simulink library "vmc"  (R2021b)
settings: Solver=VariableStepAuto  StartTime=0.0  StopTime=10.0  RelTol=1e-3
undefined symbols (not defined in the file or in its folder): AVMC_ACCDeltaTqIGain4OVRD_X_kph, AVMC_ACCDeltaTqIGain4OVRD_Y_mps2, AVMC_ACCDeltaTqIGain_X_kph, AVMC_ACCDeltaTqIGain_Y_mps2, AVMC_ACCDeltaTqPGain_X_kph, AVMC_ACCDeltaTqPGain_Y_kph, AVMC_ACCLongSteadyCtrl_X_kph, AVMC_ADSPosGFBDeltaTq_X_kph, AVMC_ADSPosGFBDeltaTq_Y_mps2, AVMC_AggressJerkPCT4AT_X_kph, AVMC_AggressJerkPCT_X_kph, AVMC_AggressLimitPCT4AT_X_kph, AVMC_AggressLimitPCT_X_kph, AVMC_CCLongSteadyCtrl_X_kph, AVMC_DISCDeltaTqIGain_X_kph, AVMC_DISCDeltaTqIGain_Y_mps2, AVMC_DISCDeltaTqPGain_X_kph, AVMC_DISCDeltaTqPGain_Y_kph, AVMC_ESCRegenOut_X_kph, AVMC_ESCRegenOut_Y_Deg, AVMC_ESCRegenOutEnSpd_X_Deg, AVMC_ISOAccLimit_X_mps, AVMC_ISODecLimit_X_mps, AVMC_ISOJerk_X_mps, AVMC_LatESCRegenOut_X_kph, AVMC_LatESCRegenOut_Y_Deg, AVMC_LongAccDeadZone_X_kph, AVMC_LongAccFiltTsforP2_X_Gps, AVMC_MCPresBaseTq_X_bar, AVMC_MSALongSteadyCtrl_X_kph, AVMC_MSAPedalOvrd_X_kph, AVMC_MSASpdBand_X_kph, AVMC_MSATqDownEndTq_X_kph, AVMC_MSATqDownTime_X_kph, AVMC_OPDDisSlideRate_X_Deg, AVMC_OVRD2ActSR2FCMCMD_X_mps2, AVMC_PedalTqRWhlRatio_X_Nm, AVMC_PedalTqRWhlRatio_Y_gps, AVMC_PedalTqRWhlSlipGain_X_rat, AVMC_PedalTqRWhlSlipGain_Y_kph, AVMC_PedalTqRWhSTRGGain_X_deg, AVMC_PedalTqRWhSTRGGain_Y_kph, AVMC_RDCDetectTime_X_kph, AVMC_RDCDetectTime_Y_pct, AVMC_RDCEnSlideRate_X_Deg, AVMC_RearWhlTqRatio_X_Nm, AVMC_RearWhlTqRatio_Y_gps, AVMC_RearWhlTqSlipGain_X_rat, AVMC_RearWhlTqSlipGain_Y_kph, AVMC_RearWhlTqSTRGGain_X_deg, AVMC_RearWhlTqSTRGGain_Y_kph, AVMC_ReqBrkJoinDecSR_X_mps2, AVMC_SoftJerkPCT_X_kph, AVMC_SoftLimitPCT_X_kph, AVMC_StESCYaw_X_kph, AVMC_StESCYaw_Y_Deg, AVMC_StESCYawCom_X_kph, AVMC_StESCYawCom_Y_Gps, AVMC_TMSpdBaseTq_X_rpm, AVMC_VehHoldDecCtrlTime2_X_kph ... (+411)
libraries: hcu_lib x108, simulink x82, tqr x1, simulink_extras x1
(part 9 of 14)

== system vmc/VMC/VMC/MSA function/MSAActivationHandshake ==
  VTQD_SpdCtrlMode_enum : Inport
  VVMC_FeatArbitrFinal_enum : Inport  Port=2
  VTQD_ExternalTqAllow_flg : Inport  Port=3
  VVMC_MeterIndSpeedForCalcu_kph : Inport  Port=4
  VVMC_FeatSetSpdFinal_raw32 : Inport  Port=5
  VTQD_SWC2CANCELSta_flg : Inport  Port=6
  VTQD_SWC2ResUpSta_flg : Inport  Port=7
  VTQD_SWC2SetdownSta_flg : Inport  Port=8
  VVMC_MSAOvrdAllow_flg : Inport  Port=9
  VINP_Distanceunit_flg : Inport  Port=10
  VTQD_GearActualPosn_enum : Inport  Port=11
  VVMC_VMCMSACtrlAvail_flg : Inport  Port=12
  VINP_SWCType_enum : Inport  Port=13
  VTQD_SWC1CANCELSta_flg : Inport  Port=14
  VTQD_SWC1ResUpSta_flg : Inport  Port=15
  VTQD_SWC1SetdownSta_flg : Inport  Port=16
  " 1" : Constant  Value=KTQD_MSAActiveMetSpdLoMPH_mph
  " 2" : Constant  Value=ENUM_SWCTYPE_SWC2
  " 80" : Constant  Value=KTQD_MSAActiveMetSpdLo_kph
  160 : Constant  Value=KTQD_MSAActiveMetSpdHi_kph
  2 : Constant  Value=KTQD_MSAActiveMetSpdHiMPH_mph
  AND : Logic  AllPortsSameDT=off  OutDataTypeStr=boolean
  AND1 : Logic  Operator=OR  AllPortsSameDT=off  OutDataTypeStr=boolean
  Cast To Boolean : DataTypeConversion  OutDataTypeStr=boolean
  Cast To Single : DataTypeConversion  OutDataTypeStr=uint8
  Cast To Single1 : DataTypeConversion  OutDataTypeStr=boolean
  Cast To Single2 : DataTypeConversion  OutDataTypeStr=single
  Cast To Single3 : DataTypeConversion  OutDataTypeStr=single
  Chart : Stateflow chart  TreatAsAtomicUnit=on
  Constant2 : Constant  Value=KVMC_CCMSASpdWar_kph
  Constant3 : Constant  Value=ENUM_ADASMSASTA_UNLIMIT
  Constant5 : Constant  Value=ENUM_FEATARBITRSTA_MSA
  Constant6 : Constant  Value=TRUE
  Constant7 : Constant  Value=FALSE
  Constant8 : Constant  Value=ENUM_ADASMSASTA_ACTIVE
  Detect Decrease2 : simulink/Logic and Bit Operations/Detect Decrease  vinit=0.0  OutDataTypeStr=boolean
  Detect Decrease3 : simulink/Logic and Bit Operations/Detect Decrease  vinit=0.0  OutDataTypeStr=boolean
  Detect Decrease4 : simulink/Logic and Bit Operations/Detect Decrease  vinit=0.0  OutDataTypeStr=boolean
  Detect Increase : simulink/Logic and Bit Operations/Detect Increase  vinit=0.0  OutDataTypeStr=boolean
  Detect Increase1 : simulink/Logic and Bit Operations/Detect Increase  vinit=0.0  OutDataTypeStr=boolean
  Detect Increase2 : simulink/Logic and Bit Operations/Detect Increase  vinit=0.0  OutDataTypeStr=boolean
  Relational Operator{,1..3} (4 alike) : RelationalOperator  Operator===  OutDataTypeStr=boolean  RndMeth=Simplest
  Switch{1..5} (5 alike) : Switch  Criteria=u2 > Threshold
  u2 > 0 : Switch  Criteria=u2 > Threshold
  VVMC_IntMSACtrlSta_enum : Outport
  VVMC_IntMSASpdWar_flg : Outport  Port=2
  VVMC_IntMSAActive_flg : Outport  Port=3
  wires:
  AND1/1 -> AND/2
  Relational Operator2/1 -> AND1/2
  Constant3/1 -> Relational Operator2/2
  [VVMC_IntMSACtrlSta_enum] -> Relational Operator2/1
  [VVMC_MSAOvrdAllow_flg] -> Chart/9(VVMC_MSAOvrdAllow_flg)
  VVMC_MSAOvrdAllow_flg/1 -> [VVMC_MSAOvrdAllow_flg]
  Cast To Single/1 -> [VVMC_IntMSACtrlSta_enum]  "VVMC_IntMSACtrlSta_enum"
  Cast To Boolean/1 -> [VVMC_IntMSAActive_flg]  "VVMC_IntMSAActive_flg"
  Cast To Single1/1 -> [VVMC_IntMSASpdWar_flg]  "VVMC_IntMSASpdWar_flg"
  VVMC_MeterIndSpeedForCalcu_kph/1 -> [VVMC_MeterIndSpeedForCalcu_kph]
  VVMC_FeatSetSpdFinal_raw32/1 -> [VVMC_FeatSetSpdFinal_raw32]
  VTQD_SWC2CANCELSta_flg/1 -> [VTQD_SWC2CANCELSta_flg]
  VTQD_ExternalTqAllow_flg/1 -> [VTQD_ExternalTqAllow_flg]
  VVMC_FeatArbitrFinal_enum/1 -> [VVMC_FeatArbitrFinal_enum]
  [VVMC_IntMSAActive_flg] -> VVMC_IntMSAActive_flg/1
  [VVMC_IntMSASpdWar_flg] -> VVMC_IntMSASpdWar_flg/1
  [VVMC_IntMSACtrlSta_enum] -> VVMC_IntMSACtrlSta_enum/1
  u2 > 0/1 -> Cast To Boolean/1
  Chart/2(VVMC_IntMSASpdWar_flg) -> Cast To Single1/1
  Chart/1(VVMC_IntMSACtrlSta_enum) -> Cast To Single/1
  Switch1/1 -> Chart/8(VVMC_DetectSWCCANCEL_flg)  "VVMC_DetectSWCCANCEL_flg"
  Constant2/1 -> Chart/7(KVMC_CCMSASpdWar_kph)
  [VVMC_FeatSetSpdFinal_raw32] -> Chart/6(VVMC_FeatSetSpdFinal_raw32)
  Switch3/1 -> Cast To Single3/1
  [VVMC_MeterIndSpeedForCalcu_kph] -> Chart/4(VVMC_MeterIndSpeedForCalcu_kph)
  Switch2/1 -> Cast To Single2/1
  [VTQD_ExternalTqAllow_flg] -> Chart/2(VTQD_ExternalTqAllow_flg)
  VTQD_SpdCtrlMode_enum/1 -> [VTQD_SpdCtrlMode_enum]
  [VTQD_SpdCtrlMode_enum] -> Chart/1(VTQD_SpdCtrlMode_enum)
  Constant8/1 -> Relational Operator1/2
  AND/1 -> u2 > 0/2
  [VVMC_FeatArbitrFinal_enum] -> Relational Operator/1
  Constant5/1 -> Relational Operator/2
  [VVMC_IntMSACtrlSta_enum] -> Relational Operator1/1
  Constant6/1 -> u2 > 0/1
  Relational Operator1/1 -> AND1/1
  Relational Operator/1 -> AND/1
  Constant7/1 -> u2 > 0/3
  Switch4/1 -> Chart/10(VVMC_DetectSWCRes_flg)  "VVMC_DetectSWCRes_flg"
  Switch5/1 -> Chart/11(VVMC_DetectSWCSet_flg)  "VVMC_DetectSWCSet_flg"
  VTQD_SWC2SetdownSta_flg/1 -> [VTQD_SWC2SetdownSta_flg]
  VTQD_SWC2ResUpSta_flg/1 -> [VTQD_SWC2ResUpSta_flg]
  [VINP_Distanceunit_flg] -> Switch2/2
  2/1 -> Switch2/1
  160/1 -> Switch2/3
  " 80"/1 -> Switch3/3
  " 1"/1 -> Switch3/1
  [VINP_Distanceunit_flg] -> Switch3/2
  VINP_Distanceunit_flg/1 -> [VINP_Distanceunit_flg]
  Cast To Single2/1 -> Chart/3(KVMC_MSAActiveMetSpdHi_kph)
  Cast To Single3/1 -> Chart/5(KVMC_MSAActiveMetSpdLo_kph)
  VTQD_GearActualPosn_enum/1 -> [VTQD_GearActualPosn_enum]
  [VTQD_GearActualPosn_enum] -> Chart/12(VTQD_GearActualPosn_enum)
  VVMC_VMCMSACtrlAvail_flg/1 -> [VVMC_VMCMSACtrlAvail_flg]
  [VVMC_VMCMSACtrlAvail_flg] -> Chart/13(VVMC_VMCMSACtrlAvail_flg)
  [VTQD_SWC2SetdownSta_flg] -> Detect Increase2/1
  [VINP_SWCType_enum] -> Relational Operator3/1
  " 2"/1 -> Relational Operator3/2
  [VTQD_SWC1SetdownSta_flg] -> Detect Decrease4/1
  Detect Increase1/1 -> Switch4/1
  [VTQD_SWC1ResUpSta_flg] -> Detect Decrease3/1
  Detect Decrease3/1 -> Switch4/3
  Detect Increase2/1 -> Switch5/1
  Detect Decrease2/1 -> Switch1/3
  [VTQD_SWC1CANCELSta_flg] -> Detect Decrease2/1
  [VTQD_SWC2CANCELSta_flg] -> Detect Increase/1
  Detect Increase/1 -> Switch1/1
  Relational Operator3/1 -> Switch5/2, Switch4/2, Switch1/2
  [VTQD_SWC2ResUpSta_flg] -> Detect Increase1/1
  Detect Decrease4/1 -> Switch5/3
  VINP_SWCType_enum/1 -> [VINP_SWCType_enum]
  VTQD_SWC1SetdownSta_flg/1 -> [VTQD_SWC1SetdownSta_flg]
  VTQD_SWC1ResUpSta_flg/1 -> [VTQD_SWC1ResUpSta_flg]
  VTQD_SWC1CANCELSta_flg/1 -> [VTQD_SWC1CANCELSta_flg]

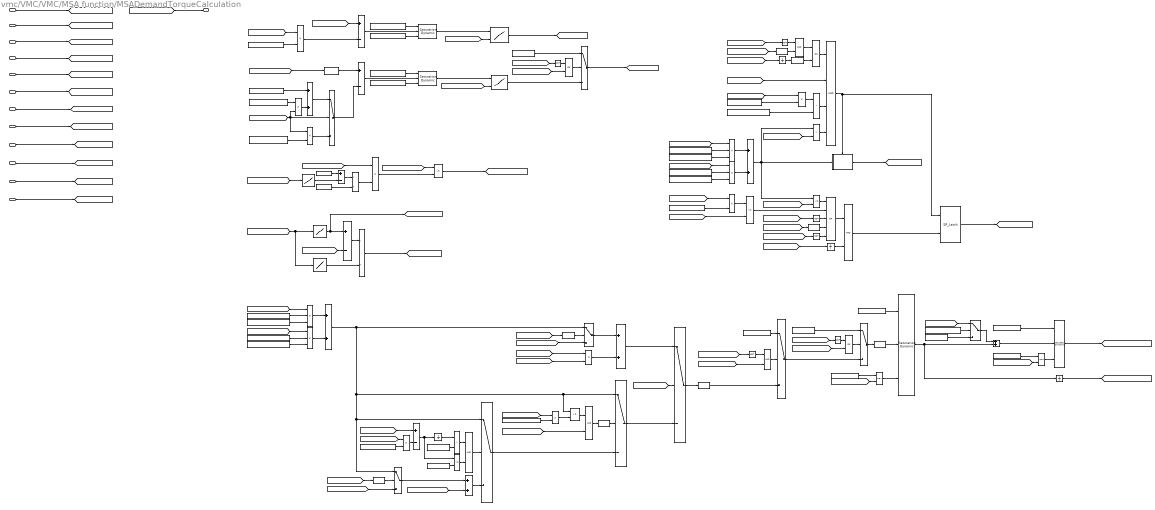
== system vmc/VMC/VMC/MSA function/MSADemandTorqueCalculation ==
  VVMC_FeatSetSpdForCalcu_kph : Inport
  VINP_VehSpeed_kph : Inport  Port=2
  VVMC_MSAActive_flg : Inport  Port=3
  VVMC_LongAcc_Gps : Inport  Port=4
  VVMC_MeterIndSpeedForCalcu_kph : Inport  Port=5
  VVMC_ActACCRequiredAccel_mps2 : Inport  Port=6
  VTQR_FrTMTqReq_Nm : Inport  Port=7
  VTQR_RrTMTqReq_Nm : Inport  Port=8
  VVMC_MSAPedalOvrd_flg : Inport  Port=9
  task_time_s : Inport  Port=10
  VTQD_LowIdleAccPedal_flg : Inport  Port=11
  VVMC_TotalAvailBrkRgnTq_Nm : Inport  Port=12
  1-D Lookup Table4 : Lookup_n-D  NumberOfTableDimensions=1  BreakpointsForDimension1=AVMC_MSASpdBand_X_kph  Table=MVMC_MSASpdBand_Y_pct  InternalRulePriority=Speed  RndMeth=Simplest  InputSameDT=on
  AND1 : Logic  Inputs=4  AllPortsSameDT=off  OutDataTypeStr=boolean
  AND2 : Logic  Operator=OR  Inputs=5  AllPortsSameDT=off  OutDataTypeStr=boolean
  AND{4..8} (5 alike) : Logic  AllPortsSameDT=off  OutDataTypeStr=boolean
  Add{,6,10,22..23} (5 alike) : Sum  Inputs=+-
  Add{1..3,5,8,12} (6 alike) : Sum
  Cast To Single4 : DataTypeConversion  OutDataTypeStr=single
  Cast To Single5 : DataTypeConversion  OutDataTypeStr=single
  Constant10 : Constant  Value=KVMC_MSATqUpLim_Nm  OutDataTypeStr=single
  Constant{18,20,31,107} (4 alike) : Constant  Value=KVMC_GravityValue_mps2
  Constant11 : Constant  Value=KVMC_MSATqUpLim_Nm  OutDataTypeStr=single
  Constant{6..7,12,41..42} (5 alike) : Constant  Value=ZERO_FLOAT
  Constant17 : Constant  Value=KVMC_MSAEnCtrlTargetAcc_mps2
  Constant2 : Constant  Value=pct
  Constant22 : Constant  Value=KTQD_RrTMTotalGearRatio_gain
  Constant23 : Constant  Value=KTQR_RrTMGearEff_c
  Constant24 : Constant  Value=KTQR_FrTMGearEff_c
  Constant25 : Constant  Value=KTQD_FrTMTotalGearRatio_gain
  Constant3 : Constant  Value=pct
  Constant32 : Constant  Value=KTQD_RrTMTotalGearRatio_gain
  Constant33 : Constant  Value=KTQR_RrTMGearEff_c
  Constant34 : Constant  Value=KTQR_FrTMGearEff_c
  Constant35 : Constant  Value=KTQD_FrTMTotalGearRatio_gain
  Constant36 : Constant  Value=KVMC_AccDevLowLim_mps2
  Constant38 : Constant  Value=KVMC_AccDevUpLim_mps2
  Constant39 : Constant  Value=KVMC_MSATqLowLim_Nm  OutDataTypeStr=single
  Constant4 : Constant  Value=KVMC_MSAPGainSW_flg
  Constant40 : Constant  Value=KVMC_MSASpdDevUpLim_kph
  Constant49 : Constant  Value=KVMC_MSATqUpLim_Nm  OutDataTypeStr=single
  Constant56 : Constant  Value=KVMC_MSASpdDevLowLim_kph
  Constant58 : Constant  Value=KVMC_Veh2MeterSpdFactor_enum
  Constant59 : Constant  Value=KVMC_Veh2MeterSpdOffset_enum
  Constant65 : Constant  Value=KVMC_Veh2MeterSpdLoFactor_enum
  Constant8 : Constant  Value=KVMC_MSATqLowLim_Nm  OutDataTypeStr=single
  Constant9 : Constant  Value=KVMC_MSATqDownEndTqRatio_pct
  Data Type Conversion1 : DataTypeConversion  OutDataTypeStr=single
  Detect Decrease1 : simulink/Logic and Bit Operations/Detect Decrease  vinit=0.0  OutDataTypeStr=boolean
  Detect Increase{,1..4} (5 alike) : simulink/Logic and Bit Operations/Detect Increase  vinit=0.0  OutDataTypeStr=boolean
  Divide : Product  Inputs=*/
  Divide{1..3,5} (4 alike) : Product  Inputs=***
  Divide{4,6,11..12} (4 alike) : Product  Inputs=**
  InitialCondition: 1 : UnitDelay  SampleTime=-1  HasFrameUpgradeWarning=on
  Logical Operator2 : Logic  Operator=OR  AllPortsSameDT=off  OutDataTypeStr=boolean
  MVMC_DISCDeltaTqIGain_Z_Nm : Lookup_n-D  BreakpointsForDimension1=AVMC_DISCDeltaTqIGain_Y_mps2  BreakpointsForDimension2=AVMC_DISCDeltaTqIGain_X_kph  Table=MVMC_DISCDeltaTqIGain_Z_Nm  InternalRulePriority=Speed  RndMeth=Simplest  InputSameDT=on
      settings: InputPortMap=u0,u1
  MVMC_DISCDeltaTqPGain_Z_Nm : Lookup_n-D  BreakpointsForDimension1=AVMC_DISCDeltaTqPGain_Y_kph  BreakpointsForDimension2=AVMC_DISCDeltaTqPGain_X_kph  BreakpointsForDimension3=[5, 7]  Table=MVMC_DISCDeltaTqPGain_Z_Nm  ExtrapMethod=Clip  InternalRulePriority=Speed  RndMeth=Simplest  InputSameDT=on
      settings: InputPortMap=u0,u1
  MVMC_MSATqDownEndTq_Y_Nm : Lookup_n-D  NumberOfTableDimensions=1  BreakpointsForDimension1=AVMC_MSATqDownEndTq_X_kph  Table=MVMC_MSATqDownEndTq_Y_Nm  InternalRulePriority=Speed  RndMeth=Simplest  InputSameDT=on
  MVMC_MSATqDownTime_Y_s : Lookup_n-D  NumberOfTableDimensions=1  BreakpointsForDimension1=AVMC_MSATqDownTime_X_kph  Table=MVMC_MSATqDownTime_Y_s  InternalRulePriority=Speed  RndMeth=Simplest  InputSameDT=on
  Max : MinMax  Function=max  Inputs=2
  Max1 : MinMax  Function=max  Inputs=2
  NOT{,1..5} (6 alike) : Logic  Operator=NOT  AllPortsSameDT=off  OutDataTypeStr=boolean
  OR : Logic  Operator=OR  AllPortsSameDT=off  OutDataTypeStr=boolean
  OR1 : Logic  Operator=OR  AllPortsSameDT=off  OutDataTypeStr=boolean
  Product{2..5,13} (5 alike) : Product
  Product14 : Product  Inputs=*/
  Relational Operator : RelationalOperator  Operator=>  OutDataTypeStr=boolean  RndMeth=Simplest
  Relational Operator1 : RelationalOperator  Operator=<=  OutDataTypeStr=boolean  RndMeth=Simplest
  Relational Operator10 : RelationalOperator  OutDataTypeStr=boolean  RndMeth=Simplest
  Relational Operator2 : RelationalOperator  Operator=>  OutDataTypeStr=boolean  RndMeth=Simplest
  Relational Operator3 : RelationalOperator  Operator=<=  OutDataTypeStr=boolean  RndMeth=Simplest
  Relational Operator4 : RelationalOperator  Operator=>  OutDataTypeStr=boolean  RndMeth=Simplest
  Relational Operator5 : RelationalOperator  Operator=<=  OutDataTypeStr=boolean  RndMeth=Simplest
  Relational Operator8 : RelationalOperator  OutDataTypeStr=boolean  RndMeth=Simplest
  SR_Latch5 : hcu_lib/Basic_Blocks/SR_Latch
  Saturation Dynamic{1,7..9} (4 alike) : simulink/Discontinuities/Saturation Dynamic  OutMin=[]  OutMax=[]  OutDataTypeStr=Inherit: Same as second input  OutDataType=fixdt(1, 16)  OutScaling=2^-10  DoSatur=off
  Switch{,2..6,8,10,12} (9 alike) : Switch  Criteria=u2 > Threshold
  Switch7 : Switch  Criteria=u2 > Threshold  Threshold=KVMC_Veh2MeterSpdLoBdy_kph
  Triggered Subsystem : Subsystem  TreatAsAtomicUnit=on
  Unit Delay : UnitDelay  SampleTime=-1  HasFrameUpgradeWarning=on
  Unit Delay2 : UnitDelay  SampleTime=-1  HasFrameUpgradeWarning=on
  Unit Delay3 : UnitDelay  SampleTime=-1  HasFrameUpgradeWarning=on
  VVMC_MSAWhlTqCal_Nm : Outport
  wires:
  [VVMC_MSAPedalOvrd_flg] -> NOT3/1
  NOT3/1 -> AND6/1
  AND6/1 -> Logical Operator2/1
  Unit Delay3/1 -> AND5/2
  [VVMC_MSATqDown_flg] -> Unit Delay3/1
  Detect Increase4/1 -> AND2/4
  NOT1/1 -> AND2/5
  [VVMC_MSAActive_flg] -> AND1/2
  AND4/1 -> Switch12/2
  Relational Operator4/1 -> AND4/1
  Relational Operator5/1 -> AND4/2
  Switch12/1 -> Switch4/3  "VVMC_MSAWhlTqCalAftGCtrl_Nm"
  Constant42/1 -> Relational Operator5/2
  Constant41/1 -> Relational Operator4/2
  Unit Delay/1 -> Relational Operator4/1
  Add10/1 -> Unit Delay/1, Relational Operator5/1
  [VVMC_LongAcc_Gps] -> Product5/1
  Constant31/1 -> Product5/2
  [VVMC_MSAReqAcc_mps2] -> Add10/1
  Product5/1 -> Add10/2
  VTQD_LowIdleAccPedal_flg/1 -> [VTQD_LowIdleAccPedal_flg]
  Relational Operator3/1 -> AND2/1
  [VVMC_MSATqDownEndTq_Nm] -> Relational Operator3/2
  [VVMC_MSAPedalOvrd_flg] -> Detect Increase4/1
  Switch/1 -> Add5/1
  [VVMC_LastMSAWhlTqCalW_Nm] -> Switch/3
  Detect Increase/1 -> Switch/2
  [VVMC_MSATqDown_flg] -> Detect Increase/1
  Logical Operator2/1 -> AND1/1
  Detect Decrease1/1 -> Logical Operator2/2
  [VVMC_MSAPedalOvrd_flg] -> Unit Delay2/1
  Unit Delay2/1 -> Detect Decrease1/1
  Divide6/1 -> Add5/2
  Add5/1 -> Switch10/1  "VVMC_MSAWhlTqCalAftTqDown_Nm"
  [task_time_s] -> Divide6/2
  [VVMC_MSATqDownSlope_Nmps] -> Divide6/1
  task_time_s/1 -> [task_time_s]
  Constant33/1 -> Divide5/3
  Divide3/1 -> Add2/1
  [VTQR_RrTMTqReq_Nm] -> Divide5/1
  Constant35/1 -> Divide3/2
  Constant32/1 -> Divide5/2
  Divide5/1 -> Add2/2
  Constant34/1 -> Divide3/3
  [VTQR_FrTMTqReq_Nm] -> Divide3/1
  [VVMC_MSATqDown_flg] -> Switch10/2
  Divide/1 -> [VVMC_MSATqDownSlope_Nmps]  "VVMC_MSATqDownSlope_Nmps"
  MVMC_MSATqDownTime_Y_s/1 -> Divide/2
  Add/1 -> Divide/1
  MVMC_MSATqDownEndTq_Y_Nm/1 -> [VVMC_MSATqDownEndTq_Nm], Add/1  "VVMC_MSATqDownEndTq_Nm"
  [VVMC_MSATqDownEnTq_Nm] -> Add/2
  [VVMC_MSATqDownEndTq_Nm] -> Relational Operator2/2
  Relational Operator2/1 -> AND1/4
  Triggered Subsystem/1(Out1) -> [VVMC_MSATqDownEnTq_Nm]  "VVMC_MSATqDownEnTq_Nm"
  SR_Latch5/1 -> [VVMC_MSATqDown_flg]  "VVMC_MSATqDown_flg"
  Relational Operator1/1 -> AND2/2
  NOT/1 -> AND2/3
  [VVMC_MSAActive_flg] -> NOT/1
  AND2/1 -> AND5/1
  Add1/1 -> Relational Operator3/1, Triggered Subsystem/1(In1), Relational Operator2/1
  [VTQR_FrTMTqReq_Nm] -> Divide1/1
  Constant24/1 -> Divide1/3
  Divide2/1 -> Add1/2
  Constant22/1 -> Divide2/2
  Constant25/1 -> Divide1/2
  [VTQR_RrTMTqReq_Nm] -> Divide2/1
  Constant23/1 -> Divide2/3
  Divide1/1 -> Add1/1
  AND1/1 -> SR_Latch5/1, Triggered Subsystem/Trigger
  Constant20/1 -> Product4/2
  [VVMC_LongAcc_Gps] -> Product4/1
  Product4/1 -> Relational Operator1/1
  [VVMC_MSAReqAcc_mps2] -> Relational Operator1/2
  Relational Operator/1 -> AND1/3
  Detect Increase2/1 -> AND6/2
  [VVMC_MSAInCtrlSpd_flg] -> Detect Increase2/1
  Constant17/1 -> Relational Operator/2
  Product3/1 -> Relational Operator/1
  [VVMC_LongAcc_Gps] -> Product3/1
  Constant18/1 -> Product3/2
  VVMC_MSAPedalOvrd_flg/1 -> [VVMC_MSAPedalOvrd_flg]
  VTQR_RrTMTqReq_Nm/1 -> [VTQR_RrTMTqReq_Nm]
  VTQR_FrTMTqReq_Nm/1 -> [VTQR_FrTMTqReq_Nm]
  VVMC_ActACCRequiredAccel_mps2/1 -> [VVMC_MSAReqAcc_mps2]
  [VVMC_FeatSetSpdForCalcu_kph] -> MVMC_DISCDeltaTqPGain_Z_Nm/2
  Switch3/1 -> Cast To Single5/1
  Saturation Dynamic9/1 -> MVMC_DISCDeltaTqPGain_Z_Nm/1
  [VVMC_MSAIGainDeltaTq_Nm] -> Add12/2
  InitialCondition: 1/1 -> [VVMC_LastMSAWhlTqCalW_Nm]  "VVMC_MSAWhlTqCalDelay_Nm"
  Add23/1 -> Saturation Dynamic9/2
  Switch6/1 -> Add12/1
  Saturation Dynamic8/1 -> MVMC_DISCDeltaTqIGain_Z_Nm/1
  Constant38/1 -> Saturation Dynamic8/1
  MVMC_DISCDeltaTqIGain_Z_Nm/1 -> [VVMC_MSAIGainDeltaTq_Nm]  "VVMC_MSAIGainDeltaTq_Nm"
  Data Type Conversion1/1 -> Add23/1
  Constant40/1 -> Saturation Dynamic9/1
  Saturation Dynamic7/1 -> InitialCondition: 1/1, Add3/2
  Add12/1 -> Switch12/3
  Constant39/1 -> Max/1
  Product2/1 -> Add22/2
  [VVMC_MSAReqAcc_mps2] -> Add22/1
  Constant107/1 -> Product2/2
  Cast To Single5/1 -> Saturation Dynamic7/2
  [VVMC_FeatSetSpdForCalcu_kph] -> Data Type Conversion1/1
  Constant36/1 -> Saturation Dynamic8/3
  [VINP_VehSpeed_kph] -> MVMC_DISCDeltaTqIGain_Z_Nm/2
  [VVMC_LongAcc_Gps] -> Product2/1
  Switch8/1 -> [VVMC_MSAPGainDeltaTq_Nm]  "VVMC_MSAPGainDeltaTq_Nm"
  Constant56/1 -> Saturation Dynamic9/3
  Switch10/1 -> Cast To Single4/1
  Add22/1 -> Saturation Dynamic8/2
  Constant49/1 -> Saturation Dynamic7/1
  VVMC_MeterIndSpeedForCalcu_kph/1 -> [VVMC_MeterIndSpeedForCalcu_kph]
  VVMC_LongAcc_Gps/1 -> [VVMC_LongAcc_Gps]
  VVMC_MSAActive_flg/1 -> [VVMC_MSAActive_flg]
  VINP_VehSpeed_kph/1 -> [VINP_VehSpeed_kph]
  VVMC_FeatSetSpdForCalcu_kph/1 -> [VVMC_FeatSetSpdForCalcu_kph]
  [VVMC_MSAWhlTqCal_Nm] -> VVMC_MSAWhlTqCal_Nm/1
  [VVMC_FeatSetSpdForCalcu_kph] -> MVMC_MSATqDownTime_Y_s/1, MVMC_MSATqDownEndTq_Y_Nm/1
  Cast To Single4/1 -> Switch5/3
  NOT4/1 -> OR/1
  [VTQD_LowIdleAccPedal_flg] -> AND7/2
  [VVMC_MSAInCtrlSpd_flg] -> AND8/2
  AND8/1 -> Detect Increase1/1
  Switch4/1 -> Switch10/3  "VVMC_MSAWhlTqCalNotTqDown_Nm"
  Add2/1 -> Switch/1, Switch6/1, Switch12/1, Relational Operator10/1, Switch4/1
  Relational Operator10/1 -> AND8/1
  [VVMC_MSATqDownEndTq_Nm] -> Divide4/1
  Detect Increase1/1 -> Switch4/2
  Divide4/1 -> Relational Operator10/2
  Constant9/1 -> Divide4/2
  [VVMC_MSAActive_flg] -> NOT4/1
  Constant6/1 -> Switch3/1
  OR/1 -> Switch3/2
  [VVMC_MSAPedalOvrd_flg] -> OR/2
  Switch5/1 -> Switch3/3  "VVMC_MSAWhlTqCalAftInCtrlSpd_Nm"
  AND7/1 -> Switch5/2
  Constant10/1 -> Switch5/1
  VVMC_TotalAvailBrkRgnTq_Nm/1 -> [VVMC_TotalAvailBrkRgnTq_Nm]
  [VVMC_TotalAvailBrkRgnTq_Nm] -> Max/2
  Max/1 -> Saturation Dynamic7/3
  [VVMC_MSAActive_flg] -> Detect Increase3/1
  Detect Increase3/1 -> Switch6/2
  [VVMC_LastMSAWhlTqCalW_Nm] -> Switch6/3
  [VVMC_FeatSetSpdForCalcu_kph] -> 1-D Lookup Table4/1
  [VVMC_MeterIndSpeedForCalcu_kph] -> Relational Operator8/1
  [VVMC_FeatSetSpdForCalcu_kph] -> Product13/1
  Constant2/1 -> Add6/1
  1-D Lookup Table4/1 -> Add6/2
  Add6/1 -> Product14/1
  Constant3/1 -> Product14/2
  Product14/1 -> Product13/2
  Product13/1 -> Relational Operator8/2
  Relational Operator8/1 -> [VVMC_MSAInCtrlSpd_flg]  "VVMC_MSAInCtrlSpd_flg"
  [VVMC_MSAInCtrlSpd_flg] -> NOT1/1
  [VVMC_MSAInCtrlSpd_flg] -> NOT2/1
  NOT2/1 -> AND7/1
  [VVMC_MSAPGainDeltaTq_Nm] -> Switch2/1
  Saturation Dynamic1/1 -> [VVMC_MSAWhlTqCal_Nm]  "VVMC_MSAWhlTqCal_Nm"
  Constant4/1 -> Switch2/2
  Constant7/1 -> Switch2/3
  Switch2/1 -> Add3/1
  Divide12/1 -> Switch7/3
  Constant65/1 -> Divide12/2
  Divide11/1 -> Add8/2
  Add8/1 -> Switch7/1
  Switch7/1 -> Add23/2
  Constant59/1 -> Add8/1
  Constant58/1 -> Divide11/1
  [VINP_VehSpeed_kph] -> Divide11/2, Switch7/2, Divide12/1
  Max1/1 -> Saturation Dynamic1/3
  [VVMC_TotalAvailBrkRgnTq_Nm] -> Max1/2
  Constant11/1 -> Saturation Dynamic1/1
  Constant8/1 -> Max1/1
  Add3/1 -> Saturation Dynamic1/2
  [VVMC_MSAPedalOvrd_flg] -> OR1/2
  OR1/1 -> Switch8/2
  Constant12/1 -> Switch8/1
  [VVMC_MSAActive_flg] -> NOT5/1
  NOT5/1 -> OR1/1
  MVMC_DISCDeltaTqPGain_Z_Nm/1 -> Switch8/3
  AND5/1 -> SR_Latch5/2

== system vmc/VMC/VMC/MSA function/MSATorqueSourceDetermination ==
  VVMC_MSAWhlTqCal_Nm : Inport
  VTQD_DriverWhlTqDem_Nm : Inport  Port=2
  VTQD_LowIdleAccPedal_flg : Inport  Port=3
  VDHP_ActAPSPosn_pct : Inport  Port=4
  VINP_VehSpeed_kph : Inport  Port=5
  task_time_s : Inport  Port=6
  VVMC_FeatSetSpdForCalcu_kph : Inport  Port=7
  VVMC_MeterIndSpeedForCalcu_kph : Inport  Port=8
  VVMC_MSAActive_flg : Inport  Port=9
  VTQD_SWCResUpSta_flg : Inport  Port=10
  VVMC_AntiSpdLimSpdEn_flg : Inport  Port=11
  1-D Lookup Table : Lookup_n-D  NumberOfTableDimensions=1  BreakpointsForDimension1=AVMC_MSASpdBand_X_kph  Table=MVMC_MSASpdBand_Y_pct  InternalRulePriority=Speed  RndMeth=Simplest  InputSameDT=on
  AND : Logic  Inputs=3  AllPortsSameDT=off  OutDataTypeStr=boolean
  Add11 : Sum  Inputs=+-
  Add2 : Sum
  Cast To Single5 : DataTypeConversion  OutDataTypeStr=single
  Constant : Constant  Value=KVMC_MSAOvrdJudgeSpd_kph
  Constant1 : Constant  Value=KVMC_MSAOvrdResAPSPosn_pct
  Constant10 : Constant  Value=TRUE
  Constant11 : Constant  Value=FALSE
  Constant13 : Constant  Value=KVMC_MSAOvrdTqRampSlope_Nmps
  Constant14 : Constant  Value=KVMC_MSATqLowLim_Nm  OutDataTypeStr=single
  Constant16 : Constant  Value=TRUE
  Constant17 : Constant  Value=FALSE
  Constant3 : Constant  Value=KVMC_MSAOvrdDetTime_s
  Constant4 : Constant  Value=KVMC_MSAOvrdResumeTime_s
  Constant43 : Constant  Value=pct
  Constant45 : Constant  Value=pct
  Constant49 : Constant  Value=KVMC_MSATqUpLim_Nm  OutDataTypeStr=single
  Detect Increase : simulink/Logic and Bit Operations/Detect Increase  vinit=0.0  OutDataTypeStr=boolean
  Detect Increase1 : simulink/Logic and Bit Operations/Detect Increase  vinit=0.0  OutDataTypeStr=boolean
  Detect Increase3 : simulink/Logic and Bit Operations/Detect Increase  vinit=0.0  OutDataTypeStr=boolean
  Divide : Product  Inputs=**
  Logical Operator : Logic  Inputs=3  AllPortsSameDT=off  OutDataTypeStr=boolean
  Logical Operator1 : Logic  Inputs=4  AllPortsSameDT=off  OutDataTypeStr=boolean
  Logical Operator2 : Logic  Operator=OR  AllPortsSameDT=off  OutDataTypeStr=boolean
  Logical Operator3 : Logic  Operator=OR  Inputs=3  AllPortsSameDT=off  OutDataTypeStr=boolean
  Logical Operator4 : Logic  Inputs=3  AllPortsSameDT=off  OutDataTypeStr=boolean
  Logical Operator5 : Logic  Operator=OR  AllPortsSameDT=off  OutDataTypeStr=boolean
  MVMC_MSAPedalOvrd_Y_pct1 : Lookup_n-D  NumberOfTableDimensions=1  BreakpointsForDimension1=AVMC_MSAPedalOvrd_X_kph  Table=MVMC_MSAPedalOvrd_Y_pct  ExtrapMethod=Clip  InternalRulePriority=Speed  RndMeth=Simplest  InputSameDT=on
  Min : MinMax  Inputs=2
  Min1 : MinMax  Inputs=2
  NOT{1..6} (6 alike) : Logic  Operator=NOT  AllPortsSameDT=off  OutDataTypeStr=boolean
  Product6 : Product
  Product7 : Product  Inputs=*/
  Relational Operator{,3,5..6} (4 alike) : RelationalOperator  OutDataTypeStr=boolean  RndMeth=Simplest
  Relational Operator1 : RelationalOperator  Operator=<=  OutDataTypeStr=boolean  RndMeth=Simplest
  Relational Operator2 : RelationalOperator  Operator=>  OutDataTypeStr=boolean  RndMeth=Simplest
  Relational Operator4 : RelationalOperator  Operator=<=  OutDataTypeStr=boolean  RndMeth=Simplest
  Relational Operator7 : RelationalOperator  Operator=>  OutDataTypeStr=boolean  RndMeth=Simplest
  Relational Operator8 : RelationalOperator  Operator=<=  OutDataTypeStr=boolean  RndMeth=Simplest
  SR_Latch1 : hcu_lib/Basic_Blocks/SR_Latch
  SR_Latch5 : hcu_lib/Basic_Blocks/SR_Latch
  Saturation Dynamic7 : simulink/Discontinuities/Saturation Dynamic  OutMin=[]  OutMax=[]  OutDataTypeStr=Inherit: Same as second input  OutDataType=fixdt(1, 16)  OutScaling=2^-10  DoSatur=off
  Switch : Switch  Criteria=u2 ~= 0
  Switch{1,3..6} (5 alike) : Switch  Criteria=u2 > Threshold
  Timer : hcu_lib/Basic_Blocks/Timer
  Timer1 : hcu_lib/Basic_Blocks/Timer
  Triggered Subsystem2 : Subsystem  TreatAsAtomicUnit=on
  Unit Delay{,1..3} (4 alike) : UnitDelay  SampleTime=-1  HasFrameUpgradeWarning=on
  VVMC_MSAWhlTqReq_Nm : Outport
  VVMC_MSAOvrdAllow_flg : Outport  Port=2
  VVMC_MSAWhlTqActive_flg : Outport  Port=3
  wires:
  Switch3/1 -> Switch1/2, Switch/2
  [VVMC_MSAWhlTqActive_flg] -> VVMC_MSAWhlTqActive_flg/1
  Switch1/1 -> [VVMC_MSAWhlTqActive_flg]  "VVMC_MSAWhlTqActive_flg"
  Constant10/1 -> Switch1/3
  Constant11/1 -> Switch1/1
  Relational Operator6/1 -> Logical Operator1/4
  Product6/1 -> Relational Operator6/2
  [VVMC_FeatSetSpdForCalcu_kph] -> Product6/1
  Constant45/1 -> Product7/2
  Product7/1 -> Product6/2
  [VVMC_MeterIndSpeedForCalcu_kph] -> Relational Operator6/1
  1-D Lookup Table/1 -> Add11/2
  Add11/1 -> Product7/1
  Constant43/1 -> Add11/1
  [VVMC_MSAActive_flg] -> NOT5/1
  NOT5/1 -> Logical Operator3/2
  [VVMC_MSAActive_flg] -> Logical Operator1/3
  NOT4/1 -> Logical Operator5/2
  [VVMC_MSAActive_flg] -> NOT4/1
  [VVMC_MSAActive_flg] -> Logical Operator/1
  VVMC_MSAActive_flg/1 -> [VVMC_MSAActive_flg]
  Timer1/1 -> Relational Operator5/1
  Constant4/1 -> Timer1/4, Relational Operator5/2
  [task_time_s] -> Timer1/3
  NOT3/1 -> Timer1/2
  [VVMC_MSAOvrdProhibit_flg] -> Logical Operator3/3
  Logical Operator3/1 -> Timer1/1, NOT3/1
  Logical Operator4/1 -> Logical Operator3/1
  VVMC_MeterIndSpeedForCalcu_kph/1 -> [VVMC_MeterIndSpeedForCalcu_kph]
  Detect Increase1/1 -> SR_Latch1/1, Triggered Subsystem2/Trigger
  Relational Operator3/1 -> Detect Increase1/1
  [VVMC_MSAOvrdAllow_flg] -> VVMC_MSAOvrdAllow_flg/1
  Timer/1 -> Relational Operator3/1
  VVMC_FeatSetSpdForCalcu_kph/1 -> [VVMC_FeatSetSpdForCalcu_kph]
  MVMC_MSAPedalOvrd_Y_pct1/1 -> Relational Operator7/2, Relational Operator2/2  "VVMC_MSAPedalOvrd_pct"
  [VVMC_MSAOvrdAllow_flg] -> Logical Operator2/1
  SR_Latch1/1 -> [VVMC_MSAOvrdAllow_flg]  "VVMC_MSAOvrdAllow_flg"
  Constant3/1 -> Timer/4, Relational Operator3/2
  [task_time_s] -> Timer/3
  task_time_s/1 -> [task_time_s]
  NOT2/1 -> Timer/2
  NOT1/1 -> Logical Operator1/2
  [VVMC_MSAOvrdProhibit_flg] -> NOT1/1
  Logical Operator1/1 -> Timer/1, NOT2/1
  [VDHP_ActAPSPosn_pct] -> Relational Operator2/1
  Switch6/1 -> [VVMC_MSAOvrdProhibit_flg]  "VVMC_MSAOvrdProhibit_flg"
  Detect Increase/1 -> Logical Operator5/1
  [VTQD_LowIdleAccPedal_flg] -> Detect Increase/1
  Relational Operator7/1 -> Logical Operator/2
  Relational Operator1/1 -> Logical Operator/3
  Constant/1 -> Relational Operator1/2
  [VINP_VehSpeed_kph] -> Relational Operator1/1
  VINP_VehSpeed_kph/1 -> [VINP_VehSpeed_kph]
  VDHP_ActAPSPosn_pct/1 -> [VDHP_ActAPSPosn_pct]
  VTQD_LowIdleAccPedal_flg/1 -> [VTQD_LowIdleAccPedal_flg]
  VTQD_DriverWhlTqDem_Nm/1 -> [VTQD_DriverWhlTqDem_Nm]
  VVMC_MSAWhlTqCal_Nm/1 -> [VVMC_MSAWhlTqCal_Nm]
  [VVMC_MSAWhlTqReq_Nm] -> VVMC_MSAWhlTqReq_Nm/1
  Switch/1 -> [VVMC_MSAWhlTqReq_Nm], Unit Delay1/1  "VVMC_MSAWhlTqReq_Nm"
  [VVMC_MSAWhlTqCal_Nm] -> Min1/1
  [VTQD_DriverWhlTqDem_Nm] -> Relational Operator/2
  Relational Operator/1 -> Logical Operator2/2
  [VVMC_MSAWhlTqCal_Nm] -> Relational Operator/1
  [VTQD_DriverWhlTqDem_Nm] -> Switch4/3
  VTQD_SWCResUpSta_flg/1 -> [VTQD_SWCResUpSta_flg]
  [VVMC_MSAWhlTqActive_flg] -> Unit Delay/1
  Unit Delay/1 -> AND/1
  [VTQD_SWCResUpSta_flg] -> AND/2
  AND/1 -> Switch3/2
  Constant17/1 -> Switch3/1
  Logical Operator2/1 -> Switch3/3
  [VVMC_FeatSetSpdForCalcu_kph] -> 1-D Lookup Table/1
  NOT6/1 -> AND/3
  [VTQD_LowIdleAccPedal_flg] -> NOT6/1
  Relational Operator2/1 -> Logical Operator1/1
  Unit Delay1/1 -> [VVMC_LastMSAWhlTqReq_Nm]
  Switch4/1 -> Switch/1
  [VVMC_MSAOvrdEnTq_Nm] -> Switch5/1
  Constant13/1 -> Divide/1
  [task_time_s] -> Divide/2
  Divide/1 -> Add2/2
  Constant14/1 -> Saturation Dynamic7/3
  Add2/1 -> Cast To Single5/1
  Constant49/1 -> Saturation Dynamic7/1
  Cast To Single5/1 -> Saturation Dynamic7/2
  Saturation Dynamic7/1 -> Min/1, Unit Delay2/1  "VVMC_MSAOvrdWhlTqCal_Nm"
  [VTQD_DriverWhlTqDem_Nm] -> Min/2
  Min/1 -> Switch4/1
  [VVMC_LastMSAWhlTqReq_Nm] -> Triggered Subsystem2/1(In1)
  Triggered Subsystem2/1(Out1) -> [VVMC_MSAOvrdEnTq_Nm]  "VVMC_MSAOvrdEnTq_Nm"
  [VVMC_MSAOvrdAllow_flg] -> Detect Increase3/1
  Detect Increase3/1 -> Switch5/2
  Switch5/1 -> Add2/1
  Unit Delay2/1 -> Switch5/3
  [VVMC_MSAOvrdAllow_flg] -> Switch4/2
  VVMC_AntiSpdLimSpdEn_flg/1 -> [VVMC_AntiSpdLimSpdEn_flg]
  [VVMC_AntiSpdLimSpdEn_flg] -> Switch6/2
  SR_Latch5/1 -> Switch6/3
  Constant16/1 -> Switch6/1
  Logical Operator5/1 -> SR_Latch5/2
  Logical Operator/1 -> SR_Latch5/1
  Min1/1 -> Switch/3
  [VTQD_DriverWhlTqDem_Nm] -> Min1/2
  Relational Operator5/1 -> SR_Latch1/2
  [VDHP_ActAPSPosn_pct] -> Relational Operator7/1
  [VVMC_FeatSetSpdForCalcu_kph] -> MVMC_MSAPedalOvrd_Y_pct1/1
  [VVMC_MSAOvrdAllow_flg] -> Unit Delay3/1
  Relational Operator4/1 -> Logical Operator4/2
  Unit Delay3/1 -> Logical Operator4/1
  [VVMC_MeterIndSpeedForCalcu_kph] -> Relational Operator8/1
  [VVMC_FeatSetSpdForCalcu_kph] -> Relational Operator8/2
  Relational Operator8/1 -> Logical Operator4/3
  [VDHP_ActAPSPosn_pct] -> Relational Operator4/1
  Constant1/1 -> Relational Operator4/2

== system vmc/VMC/VMC/RDC Determination/RWD ==
  task_time_s : Inport
  VVMC_ActMaxSlideRate_pct : Inport  Port=2
  VTQD_AfterAvailableTqDemFr_Nm : Inport  Port=3
  VTQD_AfterAvailableTqDemRr_Nm : Inport  Port=4
  VINP_ESCActive_flg : Inport  Port=5
  VINP_SASAngle_Deg : Inport  Port=6
  VINP_LatAccel_Gps : Inport  Port=7
  VINP_VehSpeed_kph : Inport  Port=8
  VINP_YawRate_degps : Inport  Port=9
  VINP_RDCActive_enum : Inport  Port=10
  VINP_DIDGetDynoMode_flg : Inport  Port=11
  AND{,2..5} (5 alike) : Logic  AllPortsSameDT=off  OutDataTypeStr=boolean
  AND1 : Logic  Inputs=3  AllPortsSameDT=off  OutDataTypeStr=boolean
  Abs{,1..7} (8 alike) : Abs
  Add1 : Sum
  Constant1 : Constant  Value=ZERO_INT
  Constant2 : Constant  Value=KVMC_DIDGetDynoModeSW_flg
  Constant{3..4,74,78} (4 alike) : Constant  Value=KVMC_AltRDCActiveTq_Nm
  Constant73 : Constant  Value=ENUM_RDCACTSTA_NOREQUEST
  Constant77 : Constant  Value=ENUM_RDCACTSTA_RAMPOUT
  Constant81 : Constant  Value=KVMC_AltRDCActiveSW_flg
  Constant82 : Constant  Value=ENUM_RDCACTSTA_EXITIMMEDIATELY
  Constant83 : Constant  Value=KVMC_AltRDCRecTime_s
  Constant86 : Constant  Value=KVMC_ESCRegenTqRecDelay_s
  Constant95 : Constant  Value=ENUM_RDCACTSTA_EXITIMMEDIATELY
  Delay{1..2,6..7} (4 alike) : Delay  DelayLength=1
  DelayEnable1 : hcu_lib/Basic_Blocks/DelayEnable
  DelayEnable2 : hcu_lib/Basic_Blocks/DelayEnable
  DelayEnable3 : hcu_lib/Basic_Blocks/DelayEnable
  Equal33 : RelationalOperator  Operator===  OutDataTypeStr=boolean  RndMeth=Simplest
  MVMC_ESCRegenOutEnSpd_Y_kph : Lookup_n-D  NumberOfTableDimensions=1  BreakpointsForDimension1=AVMC_ESCRegenOutEnSpd_X_Deg  Table=MVMC_ESCRegenOutEnSpd_Y_kph  ExtrapMethod=Clip  InternalRulePriority=Speed  RndMeth=Simplest  InputSameDT=on
  MVMC_ESCRegenOut_Z_Dps : Lookup_n-D  BreakpointsForDimension1=AVMC_ESCRegenOut_Y_Deg  BreakpointsForDimension2=AVMC_ESCRegenOut_X_kph  Table=MVMC_ESCRegenOut_Z_Dps  ExtrapMethod=Clip  InternalRulePriority=Speed  RndMeth=Simplest  InputSameDT=on
      settings: InputPortMap=u0,u1
  MVMC_LatESCRegenOut_Z_Gps : Lookup_n-D  BreakpointsForDimension1=AVMC_LatESCRegenOut_Y_Deg  BreakpointsForDimension2=AVMC_LatESCRegenOut_X_kph  Table=MVMC_LatESCRegenOut_Z_Gps  ExtrapMethod=Clip  InternalRulePriority=Speed  RndMeth=Simplest  InputSameDT=on
      settings: InputPortMap=u0,u1
  MVMC_RDCDetectTime_Z_s : Lookup_n-D  BreakpointsForDimension1=AVMC_RDCDetectTime_Y_pct  BreakpointsForDimension2=AVMC_RDCDetectTime_X_kph  Table=MVMC_RDCDetectTime_Z_s  ExtrapMethod=Clip  InternalRulePriority=Speed  RndMeth=Simplest  InputSameDT=on
      settings: InputPortMap=u0,u1
  MVMC_RDCEnSlideRate_Y_pct : Lookup_n-D  NumberOfTableDimensions=1  BreakpointsForDimension1=AVMC_RDCEnSlideRate_X_Deg  Table=MVMC_RDCEnSlideRate_Y_pct  ExtrapMethod=Clip  InternalRulePriority=Speed  RndMeth=Simplest  InputSameDT=on
  MVMC_StESCYawCom_Z_Dps : Lookup_n-D  BreakpointsForDimension1=AVMC_StESCYawCom_Y_Gps  BreakpointsForDimension2=AVMC_StESCYawCom_X_kph  Table=MVMC_StESCYawCom_Z_Dps  ExtrapMethod=Clip  InternalRulePriority=Speed  RndMeth=Simplest  InputSameDT=on
      settings: InputPortMap=u0,u1
  MVMC_StESCYaw_Z_Dps : Lookup_n-D  BreakpointsForDimension1=AVMC_StESCYaw_Y_Deg  BreakpointsForDimension2=AVMC_StESCYaw_X_kph  Table=MVMC_StESCYaw_Z_Dps  ExtrapMethod=Clip  InternalRulePriority=Speed  RndMeth=Simplest  InputSameDT=on
      settings: InputPortMap=u0,u1
  NOT : Logic  Operator=NOT  AllPortsSameDT=off  OutDataTypeStr=boolean
  NOT1 : Logic  Operator=NOT  AllPortsSameDT=off  OutDataTypeStr=boolean
  NOT3 : Logic  Operator=NOT  AllPortsSameDT=off  OutDataTypeStr=boolean
  OR{,1..4,9} (6 alike) : Logic  Operator=OR  AllPortsSameDT=off  OutDataTypeStr=boolean
  OR8 : Logic  AllPortsSameDT=off  OutDataTypeStr=boolean
  Relational Operator{1,8..10} (4 alike) : RelationalOperator  OutDataTypeStr=boolean  RndMeth=Simplest
  Relational Operator{2..7} (6 alike) : RelationalOperator  Operator=<=  OutDataTypeStr=boolean  RndMeth=Simplest
  SR_Latch4 : hcu_lib/Basic_Blocks/SR_Latch
  SR_Latch5 : hcu_lib/Basic_Blocks/SR_Latch
  Switch10 : Switch  Criteria=u2 > Threshold
  Switch11 : Switch  Criteria=u2 > Threshold
  Switch8 : Switch  Criteria=u2 > Threshold
  VVMC_RWDRDCActive_enum : Outport
  VVMC_RDCEnSlideRate_pct : Outport  Port=2
  VVMC_ActStESCYaw_Dps : Outport  Port=3
  wires:
  [VVMC_RDCDetectTime_s] -> DelayEnable1/2
  MVMC_RDCEnSlideRate_Y_pct/1 -> VVMC_RDCEnSlideRate_pct/1, [VVMC_RDCEnSlideRate_pct]  "VVMC_RDCEnSlideRate_pct"
  VINP_YawRate_degps/1 -> [VINP_YawRate_degps]
  [VINP_ESCActive_flg] -> NOT1/1
  VINP_ESCActive_flg/1 -> [VINP_ESCActive_flg]
  OR2/1 -> AND3/1
  Constant73/1 -> Switch8/3
  Delay7/1 -> Relational Operator3/1
  VINP_LatAccel_Gps/1 -> [VINP_LatAccel_Gps]
  [VVMC_RDCEnSlideRate_pct] -> Relational Operator1/2
  Switch11/1 -> [VVMC_AltRDCActive_enum]  "VVMC_AltRDCActive_enum"
  VINP_VehSpeed_kph/1 -> [VINP_VehSpeed_kph]
  Constant78/1 -> Relational Operator3/2
  [VINP_SASAngle_Deg] -> Abs7/1
  VVMC_ActMaxSlideRate_pct/1 -> [VVMC_ActMaxSlideRate_pct]
  DelayEnable2/1 -> OR3/2  "VVMC_AltRDCRec_flg"
  [task_time_s] -> DelayEnable1/3
  OR9/1 -> AND4/1
  [VINP_SASAngle_Deg] -> MVMC_LatESCRegenOut_Z_Gps/1
  [VVMC_ActMaxSlideRate_pct] -> MVMC_RDCDetectTime_Z_s/1
  [VINP_LatAccel_Gps] -> Abs5/1
  VTQD_AfterAvailableTqDemRr_Nm/1 -> [VTQD_AfterAvailableTqDemRr_Nm]
  SR_Latch5/1 -> [VVMC_ESCActive_flg]  "VVMC_ESCActive_flg"
  Abs4/1 -> Relational Operator8/1
  DelayEnable1/1 -> SR_Latch4/1  "VVMC_RDCDetectEn_flg"
  Relational Operator8/1 -> OR9/2
  Constant74/1 -> Relational Operator2/2
  [VVMC_ESCSlip_flg] -> SR_Latch5/1
  Abs5/1 -> Relational Operator10/1
  [VINP_SASAngle_Deg] -> MVMC_ESCRegenOut_Z_Dps/1
  [VINP_VehSpeed_kph] -> Relational Operator9/1
  Switch8/1 -> Switch11/3
  NOT3/1 -> OR8/1
  [VTQD_AfterAvailableTqDemFr_Nm] -> Delay6/1
  Delay6/1 -> Relational Operator2/1
  MVMC_RDCDetectTime_Z_s/1 -> [VVMC_RDCDetectTime_s]  "VVMC_RDCDetectTime_s"
  [VTQD_AfterAvailableTqDemRr_Nm] -> Delay7/1
  [VINP_SASAngle_Deg] -> MVMC_RDCEnSlideRate_Y_pct/1
  AND3/1 -> DelayEnable1/1
  [VVMC_ESCActive_flg] -> OR4/1
  Relational Operator3/1 -> OR2/2
  Relational Operator9/1 -> AND4/2, AND1/1
  Relational Operator1/1 -> AND3/2
  MVMC_ESCRegenOut_Z_Dps/1 -> Relational Operator8/2  "VVMC_ESCRegenOut_Dps"
  [VINP_YawRate_degps] -> Abs4/1
  SR_Latch4/1 -> Switch8/2
  [VVMC_ActMaxSlideRate_pct] -> Abs2/1
  Switch10/1 -> VVMC_RWDRDCActive_enum/1  "VVMC_RWDRDCActive_enum"
  [VINP_RDCActive_enum] -> Equal33/1
  VINP_SASAngle_Deg/1 -> [VINP_SASAngle_Deg]
  [task_time_s] -> DelayEnable3/3
  Abs2/1 -> Relational Operator1/1
  MVMC_LatESCRegenOut_Z_Gps/1 -> Relational Operator10/2  "VVMC_LatESCRegenOut_Gps"
  NOT1/1 -> OR8/2
  Equal33/1 -> OR4/2
  [VINP_VehSpeed_kph] -> MVMC_LatESCRegenOut_Z_Gps/2
  [VVMC_ESCSlip_flg] -> NOT3/1
  Relational Operator2/1 -> OR2/1
  Relational Operator10/1 -> OR9/1
  Constant95/1 -> Switch11/1
  [VINP_VehSpeed_kph] -> MVMC_ESCRegenOut_Z_Dps/2
  OR8/1 -> DelayEnable3/1
  OR4/1 -> Switch11/2
  [VVMC_AltRDCActive_enum] -> Switch10/1
  DelayEnable3/1 -> SR_Latch5/2
  Constant77/1 -> Switch8/1
  Constant86/1 -> DelayEnable3/2
  Constant82/1 -> Equal33/2
  VTQD_AfterAvailableTqDemFr_Nm/1 -> [VTQD_AfterAvailableTqDemFr_Nm]
  VINP_RDCActive_enum/1 -> [VINP_RDCActive_enum]
  task_time_s/1 -> [task_time_s]
  Constant1/1 -> Switch10/3
  [VINP_LatAccel_Gps] -> Abs1/1
  [VINP_SASAngle_Deg] -> Abs/1
  Abs/1 -> MVMC_StESCYaw_Z_Dps/1
  Add1/1 -> VVMC_ActStESCYaw_Dps/1, [VVMC_ActStESCYaw_Dps]  "VVMC_ActStESCYaw_Dps"
  MVMC_StESCYaw_Z_Dps/1 -> Add1/1  "VVMC_StESCYaw_Dps"
  [VINP_VehSpeed_kph] -> MVMC_StESCYaw_Z_Dps/2
  [VINP_VehSpeed_kph] -> MVMC_StESCYawCom_Z_Dps/2
  MVMC_StESCYawCom_Z_Dps/1 -> Add1/2  "VVMC_StESCYawCom_Dps"
  Abs1/1 -> MVMC_StESCYawCom_Z_Dps/1
  [VINP_VehSpeed_kph] -> MVMC_RDCDetectTime_Z_s/2
  AND/1 -> DelayEnable2/1
  [task_time_s] -> DelayEnable2/3
  Relational Operator4/1 -> AND/1
  [VVMC_ActStESCYaw_Dps] -> Relational Operator6/2
  [VVMC_RDCEnSlideRate_pct] -> Relational Operator4/2
  Abs6/1 -> Relational Operator6/1
  Relational Operator6/1 -> AND/2
  Abs3/1 -> Relational Operator4/1
  [VVMC_ActMaxSlideRate_pct] -> Abs3/1
  Constant83/1 -> DelayEnable2/2
  [VINP_YawRate_degps] -> Abs6/1
  Abs7/1 -> MVMC_ESCRegenOutEnSpd_Y_kph/1
  MVMC_ESCRegenOutEnSpd_Y_kph/1 -> Relational Operator9/2  "VVMC_ESCRegenOutEnSpd_kph"
  Constant4/1 -> Relational Operator7/2
  Delay1/1 -> Relational Operator5/1
  [VTQD_AfterAvailableTqDemRr_Nm] -> Delay2/1
  Constant3/1 -> Relational Operator5/2
  Delay2/1 -> Relational Operator7/1
  Relational Operator7/1 -> OR1/2
  Relational Operator5/1 -> OR1/1
  [VTQD_AfterAvailableTqDemFr_Nm] -> Delay1/1
  OR1/1 -> AND1/3
  [VINP_ESCActive_flg] -> AND1/2
  AND4/1 -> OR/1
  AND1/1 -> OR/2
  OR/1 -> [VVMC_ESCSlip_flg]  "VVMC_ESCSlip_flg"
  Constant81/1 -> AND2/1
  AND2/1 -> Switch10/2
  VINP_DIDGetDynoMode_flg/1 -> [VINP_DIDGetDynoMode_flg]
  [VINP_DIDGetDynoMode_flg] -> AND5/1
  Constant2/1 -> AND5/2
  AND5/1 -> NOT/1
  NOT/1 -> AND2/2
  [VINP_ESCActive_flg] -> OR3/1
  OR3/1 -> SR_Latch4/2

== system vmc/VMC/VMC/SPD2ACC/ISO22179 ==
  VVMC_VehSpeed_mps : Inport
  VVMC_LimitPCT_pct : Inport  Port=2
  VDSC_PreACC_flg : Inport  Port=3
  VDSC_DISCSta_enum : Inport  Port=4
  VDSC_AutoTurnMode_flg : Inport  Port=5
  VDSC_AccDecResp_flg : Inport  Port=6
  AND : Logic  AllPortsSameDT=off  OutDataTypeStr=boolean
  AND1 : Logic  Inputs=3  AllPortsSameDT=off  OutDataTypeStr=boolean
  AND2 : Logic  Inputs=3  AllPortsSameDT=off  OutDataTypeStr=boolean
  AND3 : Logic  Inputs=3  AllPortsSameDT=off  OutDataTypeStr=boolean
  Constant : Constant  Value=pct
  Constant1 : Constant  Value=MINUSONE_FLOAT
  Constant2 : Constant  Value=KVMC_DISCDecCtrlTest_flg
  Constant3 : Constant  Value=ENUM_DISCSTA_ACTIVE
  Constant4 : Constant  Value=KVMC_DISCDecCtrlJerk_mps3
  Constant5 : Constant  Value=KVMC_AutoTurnLimitHiGain_pct
  Constant6 : Constant  Value=KVMC_AutoTurnJerkHiGain_pct
  Constant7 : Constant  Value=KVMC_DISCDecCtrlLimit_mps2
  Constant8 : Constant  Value=KVMC_AutoTurnLimitHiGain_pct
  Constant9 : Constant  Value=KVMC_DISCAccCtrlLimit_mps2
  Divide{,1,3..6} (6 alike) : Product  Inputs=**
  Divide2 : Product  Inputs=*/
  MVMC_ISOAccLimit_Y_mps2 : Lookup_n-D  NumberOfTableDimensions=1  BreakpointsForDimension1=AVMC_ISOAccLimit_X_mps  UseOneInputPortForAllInputData=on  Table=MVMC_ISOAccLimit_Y_mps2  UseLastTableValue=on  InternalRulePriority=Speed  RndMeth=Simplest  InputSameDT=on
  MVMC_ISODecLimit_Y_mps2 : Lookup_n-D  NumberOfTableDimensions=1  BreakpointsForDimension1=AVMC_ISODecLimit_X_mps  UseOneInputPortForAllInputData=on  Table=MVMC_ISODecLimit_Y_mps2  UseLastTableValue=on  InternalRulePriority=Speed  RndMeth=Simplest  InputSameDT=on
  MVMC_ISOJerk_Y_mps3 : Lookup_n-D  NumberOfTableDimensions=1  BreakpointsForDimension1=AVMC_ISOJerk_X_mps  UseOneInputPortForAllInputData=on  Table=MVMC_ISOJerk_Y_mps3  UseLastTableValue=on  InternalRulePriority=Speed  RndMeth=Simplest  InputSameDT=on
  OR : Logic  Operator=OR  Inputs=3  AllPortsSameDT=off  OutDataTypeStr=boolean
  Relational Operator : RelationalOperator  Operator===  OutDataTypeStr=boolean  RndMeth=Simplest
  Switch{,1..5} (6 alike) : Switch  Criteria=u2 > Threshold
  VVMC_ISOAccLimit_mps2 : Outport
  VVMC_ISODecLimit_mps2 : Outport  Port=2
  VVMC_ISOJerkLimit_mps3 : Outport  Port=3
  wires:
  Constant1/1 -> Divide3/1
  [VVMC_ISOJerkLimit_mps3] -> VVMC_ISOJerkLimit_mps3/1  "VVMC_ISOJerkLimit_mps3"
  [VVMC_ISODecLimit_mps2] -> VVMC_ISODecLimit_mps2/1  "VVMC_ISODecLimit_mps2"
  [VVMC_ISOAccLimit_mps2] -> VVMC_ISOAccLimit_mps2/1  "VVMC_ISOAccLimit_mps2"
  [VVMC_VehSpeed_mps] -> MVMC_ISOJerk_Y_mps3/1
  Constant/1 -> Divide2/2
  [VVMC_LimitPCT_pct] -> Divide2/1
  VVMC_LimitPCT_pct/1 -> [VVMC_LimitPCT_pct]
  VVMC_VehSpeed_mps/1 -> [VVMC_VehSpeed_mps]
  Divide/1 -> Switch2/3
  MVMC_ISOJerk_Y_mps3/1 -> Switch/3
  MVMC_ISOAccLimit_Y_mps2/1 -> Divide/2
  [VVMC_VehSpeed_mps] -> MVMC_ISODecLimit_Y_mps2/1
  Divide3/1 -> Divide1/1
  Divide2/1 -> Divide/1, Divide1/2
  MVMC_ISODecLimit_Y_mps2/1 -> Divide3/2
  [VVMC_VehSpeed_mps] -> MVMC_ISOAccLimit_Y_mps2/1
  VDSC_AccDecResp_flg/1 -> [VDSC_AccDecResp_flg]
  VDSC_PreACC_flg/1 -> [VDSC_PreACC_flg]
  VDSC_AutoTurnMode_flg/1 -> [VDSC_AutoTurnMode_flg]
  VDSC_DISCSta_enum/1 -> [VDSC_DISCSta_enum]
  Constant5/1 -> Divide5/1
  Switch1/1 -> Divide5/2, Switch4/3
  [VDSC_AccDecResp_flg] -> AND3/1
  Divide5/1 -> Switch4/1
  [VDSC_AutoTurnMode_flg] -> AND3/2
  AND3/1 -> Switch4/2
  Constant7/1 -> Switch1/1
  Divide1/1 -> Switch1/3
  [VVMC_DISCDecCtrl_flg] -> AND3/3
  [VVMC_DISCDecCtrl_flg] -> Switch1/2
  Switch4/1 -> [VVMC_ISODecLimit_mps2]
  [VVMC_DISCDecCtrl_flg] -> AND2/3
  [VDSC_AccDecResp_flg] -> AND2/1
  Constant2/1 -> AND/2
  Relational Operator/1 -> OR/2
  AND2/1 -> Switch3/2
  [VDSC_AutoTurnMode_flg] -> AND2/2
  Switch/1 -> Divide4/2, Switch3/3
  [VDSC_DISCSta_enum] -> Relational Operator/1
  Constant3/1 -> Relational Operator/2
  Divide4/1 -> Switch3/1
  Constant6/1 -> Divide4/1
  OR/1 -> AND/1
  [VDSC_AutoTurnMode_flg] -> OR/3
  Constant4/1 -> Switch/1
  AND/1 -> Switch/2, [VVMC_DISCDecCtrl_flg]  "VVMC_DISCDecCtrl_flg"
  [VDSC_PreACC_flg] -> OR/1
  Switch3/1 -> [VVMC_ISOJerkLimit_mps3]
  [VVMC_DISCDecCtrl_flg] -> Switch2/2
  [VVMC_DISCDecCtrl_flg] -> AND1/3
  Constant9/1 -> Switch2/1
  AND1/1 -> Switch5/2
  [VDSC_AutoTurnMode_flg] -> AND1/2
  Divide6/1 -> Switch5/1
  [VDSC_AccDecResp_flg] -> AND1/1
  Switch2/1 -> Divide6/2, Switch5/3
  Constant8/1 -> Divide6/1
  Switch5/1 -> [VVMC_ISOAccLimit_mps2]

== system vmc/VMC/VMC/SPD2ACC/PID ==
  VVMC_SPD2ACCAct_flg : Inport
  VVMC_FeatReqSpd_kph : Inport  Port=2
  VINP_VehSpeed_kph : Inport  Port=3
  VVMC_MeterIndSpeedForCalcu_kph : Inport  Port=4
  task_time_s : Inport  Port=5
  Cast To Single : DataTypeConversion  OutDataTypeStr=single
  Constant10 : Constant  Value=ONE_FLOAT
  Constant2 : Constant  Value=KPH2MPS
  Constant3 : Constant  Value=KPH2MPS
  Constant4 : Constant  Value=ZERO_FLOAT
  Constant5 : Constant  Value=KVMC_PParm_enum
  Constant6 : Constant  Value=KVMC_IParm_enum
  Constant8 : Constant  Value=ZERO_FLOAT
  Constant9 : Constant  Value=KVMC_AccelIGain_enum
  Divide : Product  Inputs=**
  Divide1 : Product  Inputs=***
  Divide3 : Product  Inputs=**/
  Divide4 : Product  Inputs=**
  InitialCondition: 0 : UnitDelay  SampleTime=-1  HasFrameUpgradeWarning=on
  Subtract : Sum
  Sum1 : Sum  Inputs=|+-
  Sum2 : Sum  Inputs=|+-
  Sum4 : Sum  Inputs=|++
  u2 > 0 : Switch  Criteria=u2 > Threshold
  u2 > 0 (2) : Switch  Criteria=u2 > Threshold
  u2 >= 0 : Switch
  VVMC_AccCalcuPID_mps2 : Outport
  VVMC_MeterSpdCalcu_mps : Outport  Port=2
  wires:
  Divide4/1 -> [VVMC_MeterSpdCalcu_mps]
  [task_time_s] -> Cast To Single/1
  Cast To Single/1 -> Divide3/3
  Sum4/1 -> Divide1/2
  Constant8/1 -> u2 > 0 (2)/3
  [VVMC_MeterIndSpeedForCalcu_kph] -> Sum1/2
  Divide/1 -> [VVMC_AccCalcuPIDPGain_mps2]  "VVMC_AccCalcuPIDPGain_mps2"
  Sum1/1 -> u2 > 0 (2)/2, Divide/1
  Constant5/1 -> Divide/2
  Subtract/1 -> Divide3/1
  Constant3/1 -> Divide4/2
  [VINP_VehSpeed_kph] -> Sum2/2
  Divide1/1 -> [VVMC_AccCalcuPIDIGain_mps2]  "VVMC_AccCalcuPIDIGain_mps2"
  u2 > 0 (2)/1 -> u2 >= 0/1
  [VVMC_SPD2ACCAct_flg] -> u2 > 0/2
  Constant6/1 -> Divide1/3
  Sum2/1 -> u2 >= 0/2, InitialCondition: 0/1, Sum4/1
  Constant4/1 -> u2 > 0/3
  InitialCondition: 0/1 -> Sum4/2
  u2 >= 0/1 -> Divide1/1
  Constant2/1 -> Divide3/2
  Constant10/1 -> u2 >= 0/3
  Constant9/1 -> u2 > 0 (2)/1
  [VVMC_FeatReqSpd_kph] -> Sum1/1
  VINP_VehSpeed_kph/1 -> [VINP_VehSpeed_kph]
  [VVMC_MeterSpdCalcu_mps] -> VVMC_MeterSpdCalcu_mps/1  "VVMC_MeterSpdCalcu_mps"
  [VVMC_AccCalcuPID_mps2] -> VVMC_AccCalcuPID_mps2/1  "VVMC_AccCalcuPID_mps2"
  VVMC_MeterIndSpeedForCalcu_kph/1 -> [VVMC_MeterIndSpeedForCalcu_kph]
  VVMC_FeatReqSpd_kph/1 -> [VVMC_FeatReqSpd_kph]
  VVMC_SPD2ACCAct_flg/1 -> [VVMC_SPD2ACCAct_flg]
  [VVMC_FeatReqSpd_kph] -> Sum2/1
  [VVMC_MeterIndSpeedForCalcu_kph] -> Divide4/1
  u2 > 0/1 -> [VVMC_AccCalcuPID_mps2]
  [VVMC_AccCalcuPIDIGain_mps2] -> Subtract/1
  [VVMC_AccCalcuPIDPGain_mps2] -> Subtract/2
  Divide3/1 -> u2 > 0/1
  task_time_s/1 -> [task_time_s]

== system vmc/VMC/VMC/SPD2ACC/SPD2ACC Active Determination ==
  VVMC_FeatArbitrSta_enum : Inport
  Constant : Constant  Value=TRUE
  Constant1 : Constant  Value=FALSE
  Constant13 : Constant  Value=ENUM_FEATARBITRSTA_DISC
  Constant2 : Constant  Value=ENUM_FEATARBITRSTA_ACCDISC
  Constant3 : Constant  Value=ENUM_FEATARBITRSTA_CC
  Constant4 : Constant  Value=ENUM_FEATARBITRSTA_MSA
  SPD2ACC Active Determination : Stateflow chart  TreatAsAtomicUnit=on
  VVMC_SPD2ACCAct_flg : Outport
  wires:
  Constant2/1 -> SPD2ACC Active Determination/5(ENUM_FEATARBITRSTA_ACCDISC)
  Constant13/1 -> SPD2ACC Active Determination/4(ENUM_FEATARBITRSTA_DISC)
  Constant1/1 -> SPD2ACC Active Determination/3(FALSE)
  Constant/1 -> SPD2ACC Active Determination/2(TURE)
  [VVMC_SPD2ACCAct_flg] -> VVMC_SPD2ACCAct_flg/1
  SPD2ACC Active Determination/1(VVMC_SPD2ACCAct_flg) -> [VVMC_SPD2ACCAct_flg]
  [VVMC_FeatArbitrSta_enum] -> SPD2ACC Active Determination/1(VVMC_FeatArbitrSta_enum)
  VVMC_FeatArbitrSta_enum/1 -> [VVMC_FeatArbitrSta_enum]
  Constant3/1 -> SPD2ACC Active Determination/6(ENUM_FEATARBITRSTA_CC)
  Constant4/1 -> SPD2ACC Active Determination/7(ENUM_FEATARBITRSTA_MSA)
